simulink model "system9"  (R2019a)
settings: Solver=ode45  StartTime=0.0  StopTime=10  FixedStep=0.005  RelTol=1e-3
values from neighbouring files (symbols this model uses):
  d_y0 = 0    [Lab2.m]
  K = 10    [Lab2.m]
  y0 = 0    [Lab2.m]
settings Model: Creator=Vasco  LastModifiedBy=Vasco

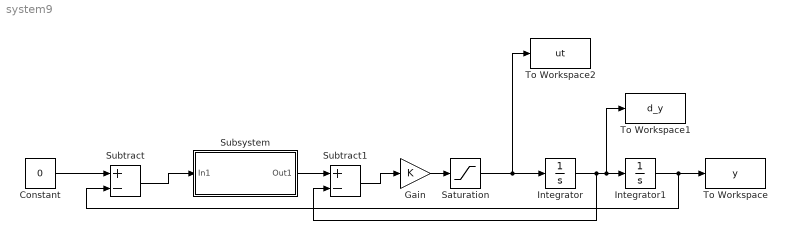
== system system9 ==
  Constant : Constant  Value=0
  Gain : Gain  Gain=K
  Integrator : Integrator  InitialCondition=d_y0
  Integrator1 : Integrator  InitialCondition=y0
  Saturation : Saturate  UpperLimit=1  LowerLimit=-1
  Subsystem : Subsystem
  Subtract : Sum  Inputs=+-
  Subtract1 : Sum  Inputs=+-
  To Workspace : ToWorkspace  VariableName=y  SampleTime=-1
      settings: Save2DSignal=2-D array (concatenate along first dimension)
  To Workspace1 : ToWorkspace  VariableName=d_y  SampleTime=-1
      settings: Save2DSignal=2-D array (concatenate along first dimension)
  To Workspace2 : ToWorkspace  VariableName=ut  SampleTime=-1
      settings: Save2DSignal=2-D array (concatenate along first dimension)
  wires:
  Gain/1 -> Saturation/1
  Saturation/1 -> To Workspace2/1, Integrator/1
  Integrator/1 -> Subtract1/2, To Workspace1/1, Integrator1/1
  Integrator1/1 -> Subtract/2, To Workspace/1
  Subtract/1 -> Subsystem/1(In1)
  Constant/1 -> Subtract/1
  Subsystem/1(Out1) -> Subtract1/1
  Subtract1/1 -> Gain/1

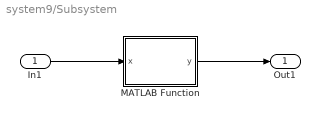
== system system9/Subsystem ==
  In1 : Inport
  MATLAB Function : MATLAB Function  TreatAsAtomicUnit=on
  Out1 : Outport
  wires:
  In1/1 -> MATLAB Function/1(x)
  MATLAB Function/1(y) -> Out1/1

== matlab function system9/Subsystem/MATLAB Function ==
  data: x input; y output
function y  = fcn(x)

    y = sign(x) * sqrt(2*abs(x));

end
